simulink model "buck_boost"  (R2025a)
settings: Solver=FixedStepAuto  StartTime=0.0  StopTime=10.0  FixedStep=0.001  RelTol=1e-3
values from neighbouring files (symbols this model uses):
  C = 470*10^-6    (= 0.00047)    [projeakt_3.m]
  E = 12    [projeakt_3.m]
  L = Ls(i)*15.91e-3    [projeakt_3.m]
  noise_var = 0    [projeakt_3.m]
  R = 52    [projeakt_3.m]
  u_eq = eval(u_eq)    [projeakt_3.m]
settings Model: Creator=PC  LastModifiedBy=PC
settings DataIOCC: ReturnWorkspaceOutputs=off

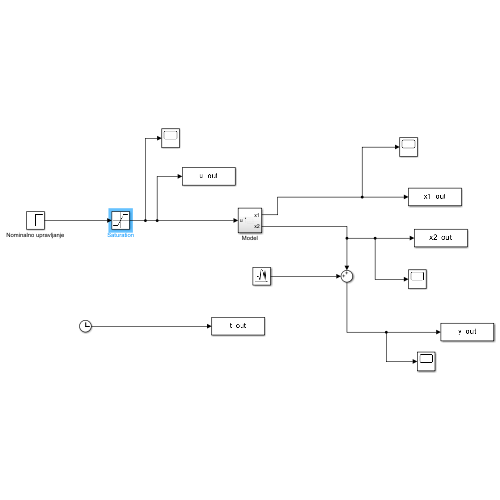
[thumbnail: Simulink's stored preview of the top-level diagram]
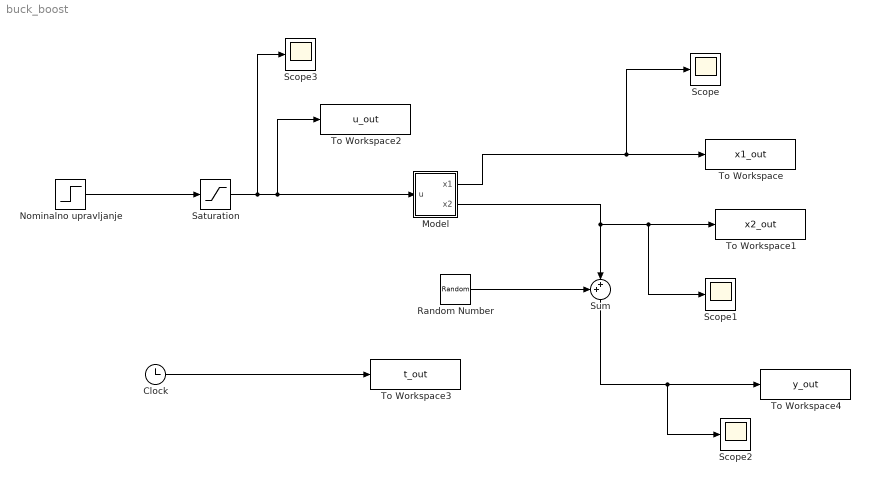
== system buck_boost ==
  Clock : Clock
  Model : Subsystem
  Nominalno upravljanje : Step  After=u_eq  SampleTime=0
  Random Number : RandomNumber  Variance=noise_var  SampleTime=0.001
  Saturation : Saturate  UpperLimit=0.90  LowerLimit=0
  Scope{,1..3} (4 alike) : Scope
      Scope settings: ActiveDisplayYMinimum=-1  ActiveDisplayYMaximum=1
      Scope1 settings: ActiveDisplayYMinimum=-1  ActiveDisplayYMaximum=1
      Scope2 settings: ActiveDisplayYMinimum=-3.9735708076417146E+227  ActiveDisplayYMaximum=-1.3645088196023411E+227  DataLoggingVariableName=ScopeData2
      Scope3 settings: ActiveDisplayYMinimum=-1  ActiveDisplayYMaximum=1  DataLoggingVariableName=ScopeData3
  Sum : Sum  Inputs=++|
  To Workspace : ToWorkspace  VariableName=x1_out  SampleTime=-1
  To Workspace1 : ToWorkspace  VariableName=x2_out  SampleTime=-1
  To Workspace2 : ToWorkspace  VariableName=u_out  SampleTime=-1
  To Workspace3 : ToWorkspace  VariableName=t_out  SampleTime=-1
  To Workspace4 : ToWorkspace  VariableName=y_out  SampleTime=-1
  wires:
  Nominalno upravljanje/1 -> Saturation/1
  Saturation/1 -> Scope3/1, To Workspace2/1, Model/1(u)
  Clock/1 -> To Workspace3/1
  Model/1(x1) -> Scope/1, To Workspace/1
  Model/2(x2) -> Sum/2, Scope1/1, To Workspace1/1
  Random Number/1 -> Sum/1
  Sum/1 -> Scope2/1, To Workspace4/1

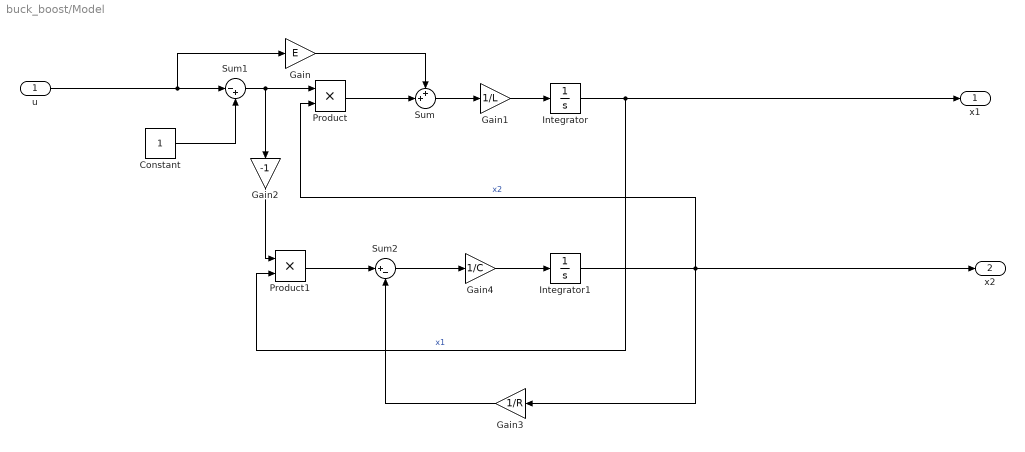
== system buck_boost/Model ==
  u : Inport
  Constant : Constant
  Gain : Gain  Gain=E
  Gain1 : Gain  Gain=1/L
  Gain2 : Gain  Gain=-1
  Gain3 : Gain  Gain=1/R
  Gain4 : Gain  Gain=1/C
  Integrator : Integrator  LimitOutput=on  LowerSaturationLimit=0
  Integrator1 : Integrator  LimitOutput=on  UpperSaturationLimit=0
  Product : Product
  Product1 : Product
  Sum : Sum  Inputs=++|
  Sum1 : Sum  Inputs=|-+
  Sum2 : Sum  Inputs=|+-
  x1 : Outport
  x2 : Outport  Port=2
  wires:
  Product1/1 -> Sum2/1
  Integrator1/1 -> x2/1, Gain3/1, Product/2  "x2"
  Gain3/1 -> Sum2/2
  Constant/1 -> Sum1/2
  Sum2/1 -> Gain4/1
  Product/1 -> Sum/2
  Gain1/1 -> Integrator/1
  Sum1/1 -> Product/1, Gain2/1
  Integrator/1 -> x1/1, Product1/2  "x1"
  Gain/1 -> Sum/1
  u/1 -> Sum1/1, Gain/1
  Gain4/1 -> Integrator1/1
  Sum/1 -> Gain1/1
  Gain2/1 -> Product1/1
